simulink model "guidance"  (R2017b)
settings: Solver=FixedStepDiscrete  StartTime=0.0  StopTime=inf  FixedStep=0.01  RelTol=1e-3
model workspace (MAT data in the model file):
  SL_ROS_VariableLengthArrays_MaxSizes.CommonInfo.ArrayTruncateAction = 'EmitWarning'
  SL_ROS_VariableLengthArrays_MaxSizes.MsgTypeMap = containers.Map
  SL_ROS_VariableLengthArrays_MaxSizes.MsgTypeMap.serialization.keys = {'sensor_msgs/Image'}
  SL_ROS_VariableLengthArrays_MaxSizes.MsgTypeMap.serialization.values{1}(1).PropertyName = 'Encoding'
  SL_ROS_VariableLengthArrays_MaxSizes.MsgTypeMap.serialization.values{1}(1).DataType = 'uint8'
  SL_ROS_VariableLengthArrays_MaxSizes.MsgTypeMap.serialization.values{1}(1).MaxLength = 128
  SL_ROS_VariableLengthArrays_MaxSizes.MsgTypeMap.serialization.values{1}(2).PropertyName = 'Data'
  SL_ROS_VariableLengthArrays_MaxSizes.MsgTypeMap.serialization.values{1}(2).DataType = 'uint8'
  SL_ROS_VariableLengthArrays_MaxSizes.MsgTypeMap.serialization.values{1}(2).MaxLength = 921600
  SL_ROS_VariableLengthArrays_MaxSizes.MsgTypeMap.serialization.uniformity = 0
  SL_ROS_VariableLengthArrays_MaxSizes.MsgTypeMap.serialization.keyType = 'char'
  SL_ROS_VariableLengthArrays_MaxSizes.MsgTypeMap.serialization.valueType = 'any'
undefined symbols (not defined in the file): Data, Data_SL_Info
libraries: dspstat3 x13, robotlib x9, simulink x7
settings Model: SimulationMode=external  Creator=a  LastModifiedBy=a
settings OptimizationCC: MaxStackSize=64
settings DebuggingCC: ParameterTunabilityLossMsg=error
settings HardwareCC: ProdBitPerPointer=32  ProdBitPerSizeT=32  ProdBitPerPtrDiffT=32  ProdLargestAtomicInteger=Long  ProdLargestAtomicFloat=Double  ProdWordSize=32  ProdHWDeviceType=ARM Compatible->ARM Cortex
settings SFSimCC: MATLABDynamicMemAlloc=off
settings RTWCC: SystemTargetFile=ert.tlc  HardwareBoard=Robot Operating System (ROS)  TemplateMakefile=ert_default_tmf  GenerateReport=on  Toolchain=Catkin  IncludeHyperlinkInReport=on  LaunchReport=on  TargetLang=C++  GenerateTraceInfo=on  GenerateTraceReport=on  GenerateTraceReportSl=on  GenerateTraceReportSf=on  GenerateTraceReportEml=on
settings CodeAppCC: ForceParamTrailComments=on  IgnoreCustomStorageClasses=off  OperatorAnnotations=on  SimulinkDataObjDesc=on  SFDataObjDesc=on  MATLABFcnDesc=on  InsertBlockDesc=on  StateflowObjectComments=on  MATLABSourceComments=on
settings ERTTargetCC: MultiwordLength=2048  ExtMode=on  ExtModeMexArgs='10.42.0.1' 0 17725
settings SimscapeCC: SimscapeNormalizeSystem=off

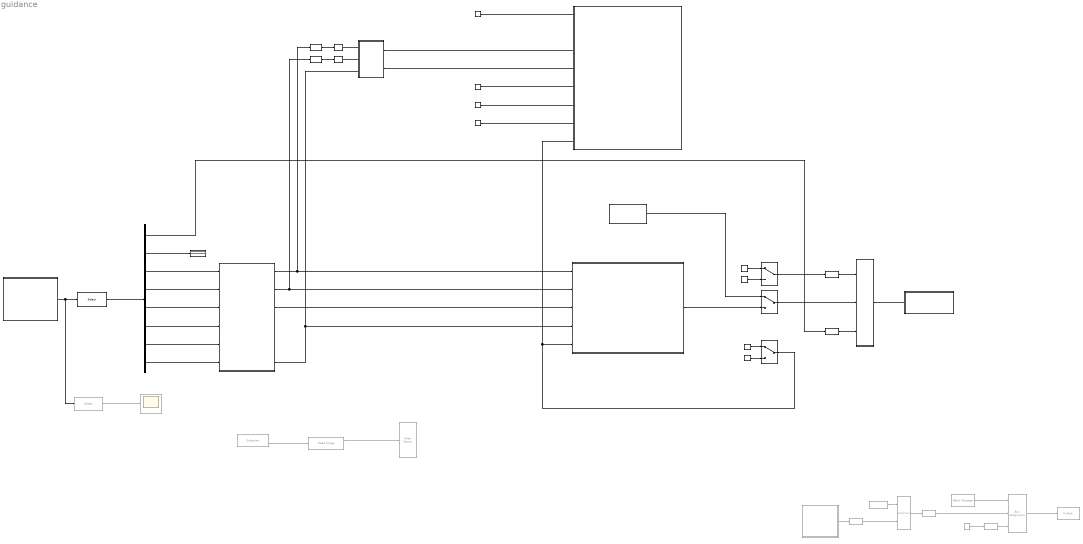
== system guidance ==
  " VX_moving_average" : dspstat3/Moving Average  Method=Sliding window  SpecifyWindowLength=on  WindowLength=5  ForgettingFactor=0.9  SimulateUsing=Code generation
  " VY_moving_average" : dspstat3/Moving Average  Method=Sliding window  SpecifyWindowLength=on  WindowLength=5  ForgettingFactor=0.9  SimulateUsing=Code generation
  Assignment : Assignment  Commented=on  DiagnosticForDimensions=Warning  IndexOptions=Index vector (dialog)  Indices=[1 2 3 4]  OutputSizes=1
  Blank Message : robotlib/Blank Message  Commented=on  SourceLibraryInfo=This block requires Robotics System Toolbox  messageType=std_msgs/Int8MultiArray  SampleTime=0.05
      settings: SourceProductBaseCode=RO
  Bus Assignment : BusAssignment  Commented=on  AssignedSignals=Data,Data_SL_Info.CurrentLength
  Constant1 : Constant  Commented=on  Value=4
  Constant3 : Constant  Commented=on  Value=[1:1:128]
  Data Type Conversion : DataTypeConversion  Commented=on  OutDataTypeStr=double
  Data Type Conversion1 : DataTypeConversion  Commented=on  OutDataTypeStr=uint32
  Data Type Conversion2 : DataTypeConversion  Commented=on  OutDataTypeStr=int8
  Data Type Conversion3 : DataTypeConversion  OutDataTypeStr=single
  Data Type Conversion4 : DataTypeConversion  OutDataTypeStr=single
  Demux : Demux  Outputs=8
  Read Image : robotlib/Read Image  Commented=on  SourceLibraryInfo=This block requires Robotics System Toolbox  MaximumImageSize=[ 320, 240 ]  ImageEncoding=rgb8  ShowAlphaOutput=off  ShowErrorCodeOutput=on  VariableSizeOutputs=off
      settings: SourceProductName=Robotics System Toolbox  SourceProductBaseCode=RO
  Scope : Scope  Commented=on
  Selector : Selector  InputPortWidth=24  IndexOptions=Index vector (dialog)  Indices=[17:24]  OutputSizes=1
  Selector1 : Selector  Commented=on  InputPortWidth=24  IndexOptions=Index vector (dialog)  Indices=[7]  OutputSizes=1
  Subscribe1 : robotlib/Subscribe  Commented=on  SourceLibraryInfo=This block requires Robotics System Toolbox  topicSource=Select from ROS network  topic=/quadrotor_1/image_raw  messageType=sensor_msgs/Image  sampleTime=-1  messageQueueLength=1
      settings: SourceProductBaseCode=RO
  Subsystem : Subsystem  Commented=on  mask{red=0.0, green=0.0, blue=15.0, enable=1}
  Video Viewer : VideoViewer  Commented=on  FigPos=[1 726 1362 626]
  X Derivative : simulink/Discrete/Discrete Derivative  gainval=1.0  ICPrevScaledInput=0.0  OutMin=[]  OutMax=[]  OutDataType=fixdt(1, 16)  OutScaling=2^-10  DoSatur=off
  Y Derivative : simulink/Discrete/Discrete Derivative  gainval=1.0  ICPrevScaledInput=0.0  OutMin=[]  OutMax=[]  OutDataType=fixdt(1, 16)  OutScaling=2^-10  DoSatur=off
  arm : Constant
  arm_disarm_sw : ManualSwitch
  check_arm_status : Subsystem
  command_output : Subsystem
  "command_output " : robotlib/Publish  Commented=on  SourceLibraryInfo=This block requires Robotics System Toolbox  topicSource=Select from ROS network  topic=/quadrotor_1/LED  messageType=std_msgs/Int8MultiArray  messageQueueLength=1
      settings: SourceProductBaseCode=RO
  "data_input " : Subsystem
  disarm : Constant  Value=0
  inertial_to_body_transform : Subsystem
  manual_auto_sw : ManualSwitch
  manual_control : Subsystem  mask{throttle=20.320, roll=0, pitch=0, yaw=0, mode=0}
  mode : Constant  Value=0
  one : Constant
  position_control : Subsystem
  position_filters : Subsystem
  radio_command_frame_rate : Display
  reset_integrator : ManualSwitch
  velocity_control : Subsystem
  vx_setpoint : Constant  Value=0
  vy_setpoint : Constant  Value=0
  yaw_des_rate : Constant  Value=0
  zero : Constant  Value=0
  wires:
  Constant1/1 -> Data Type Conversion1/1
  Data Type Conversion1/1 -> Bus Assignment/3
  Bus Assignment/1 -> "command_output "/1
  Blank Message/1 -> Bus Assignment/1
  Data Type Conversion2/1 -> Bus Assignment/2
  Assignment/1 -> Data Type Conversion2/1
  Data Type Conversion/1 -> Assignment/2
  Constant3/1 -> Assignment/1
  Subsystem/1(Out1) -> Data Type Conversion/1
  disarm/1 -> arm_disarm_sw/1
  check_arm_status/1(Out) -> command_output/1(command)
  Data Type Conversion3/1 -> check_arm_status/3(motors_on)
  Data Type Conversion4/1 -> check_arm_status/1(arm)
  manual_control/1(commands) -> manual_auto_sw/1
  manual_auto_sw/1 -> check_arm_status/2(command)
  arm/1 -> arm_disarm_sw/2
  arm_disarm_sw/1 -> Data Type Conversion4/1
  reset_integrator/1 -> velocity_control/8(Integrator_reset), position_control/5(integrator_reset)
  one/1 -> reset_integrator/2
  zero/1 -> reset_integrator/1
  "data_input "/1(data) -> Selector1/1, Selector/1
  Selector/1 -> Demux/1
  Demux/1 -> Data Type Conversion3/1
  Demux/2 -> radio_command_frame_rate/1
  Subscribe1/2 -> Read Image/1
  Read Image/1 -> Video Viewer/1
  mode/1 -> velocity_control/1(mode)
  Demux/5 -> position_filters/3(z)
  vy_setpoint/1 -> velocity_control/6(vy_setpoint)
  vx_setpoint/1 -> velocity_control/7(vx_setpoint)
  Y Derivative/1 -> " VY_moving_average"/1
  X Derivative/1 -> " VX_moving_average"/1
  Selector1/1 -> Scope/1
  position_filters/1(x_filtered) -> X Derivative/1, position_control/1(X)
  position_filters/6(psi_filtered) -> inertial_to_body_transform/3(PSI), position_control/4(PSI)
  position_filters/2(y_filtered) -> Y Derivative/1, position_control/2(Y)
  Demux/3 -> position_filters/1(x)
  Demux/4 -> position_filters/2(y)
  Demux/6 -> position_filters/4(phi)
  Demux/7 -> position_filters/5(theta)
  Demux/8 -> position_filters/6(psi)
  position_filters/3(z_filtered) -> position_control/3(Z)
  inertial_to_body_transform/1(vx) -> velocity_control/3(vx)
  inertial_to_body_transform/2(vy) -> velocity_control/4(vy)
  " VX_moving_average"/1 -> inertial_to_body_transform/1(VX)
  " VY_moving_average"/1 -> inertial_to_body_transform/2(VY)
  position_control/1(radio_command) -> manual_auto_sw/2
  yaw_des_rate/1 -> velocity_control/5(yaw_des_rate)

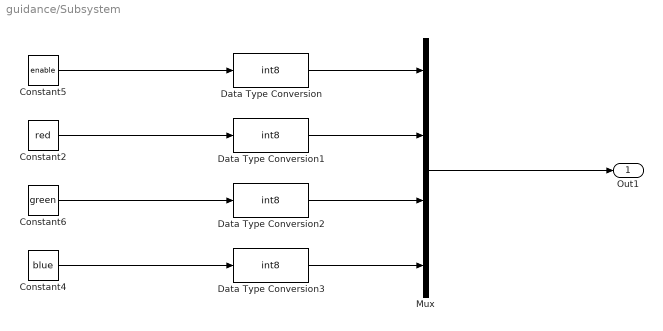
== system guidance/Subsystem ==
  Constant2 : Constant  Value=red
  Constant4 : Constant  Value=blue
  Constant5 : Constant  Value=enable
  Constant6 : Constant  Value=green
  Data Type Conversion{,1..3} (4 alike) : DataTypeConversion  OutDataTypeStr=int8
  Mux : Mux
  Out1 : Outport
  wires:
  Constant2/1 -> Data Type Conversion1/1
  Mux/1 -> Out1/1
  Constant5/1 -> Data Type Conversion/1
  Constant4/1 -> Data Type Conversion3/1
  Constant6/1 -> Data Type Conversion2/1
  Data Type Conversion/1 -> Mux/1
  Data Type Conversion1/1 -> Mux/2
  Data Type Conversion2/1 -> Mux/3
  Data Type Conversion3/1 -> Mux/4

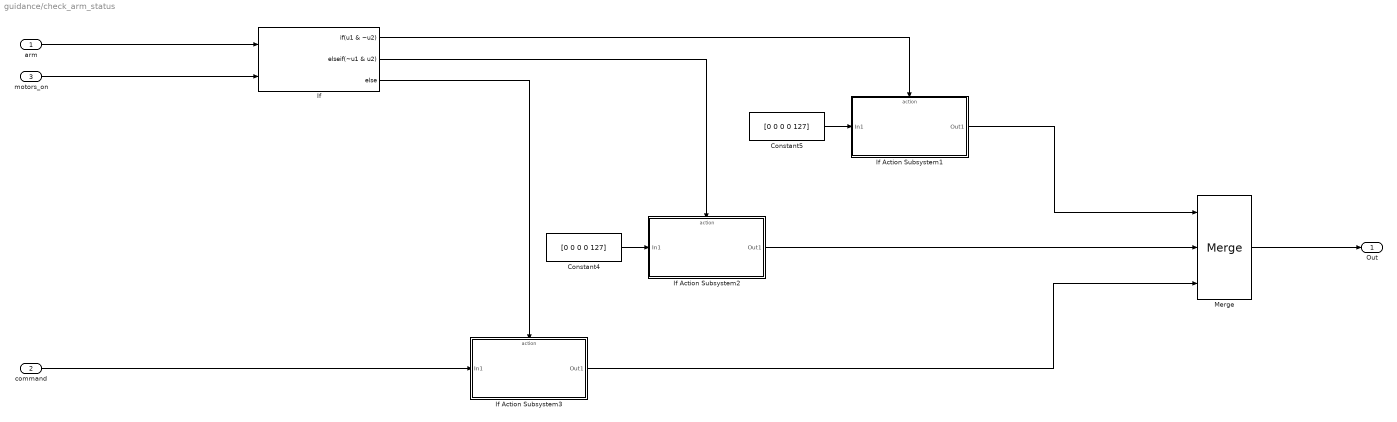
== system guidance/check_arm_status ==
  arm : Inport
  command : Inport  Port=2
  motors_on : Inport  Port=3
  Constant4 : Constant  Value=[0 0 0 0 127]
  Constant5 : Constant  Value=[0 0 0 0 127]
  If : If  NumInputs=2  IfExpression=u1 & ~u2  ElseIfExpressions=~u1 & u2
  If Action Subsystem1 : Subsystem  TreatAsAtomicUnit=on
  If Action Subsystem2 : Subsystem  TreatAsAtomicUnit=on
  If Action Subsystem3 : Subsystem  TreatAsAtomicUnit=on
  Merge : Merge  Inputs=3
  Out : Outport
  wires:
  If/1 -> If Action Subsystem1/Action
  Constant4/1 -> If Action Subsystem2/1(In1)
  If/3 -> If Action Subsystem3/Action
  Constant5/1 -> If Action Subsystem1/1(In1)
  If/2 -> If Action Subsystem2/Action
  If Action Subsystem2/1(Out1) -> Merge/2
  motors_on/1 -> If/2
  command/1 -> If Action Subsystem3/1(In1)
  If Action Subsystem1/1(Out1) -> Merge/1
  If Action Subsystem3/1(Out1) -> Merge/3
  arm/1 -> If/1
  Merge/1 -> Out/1

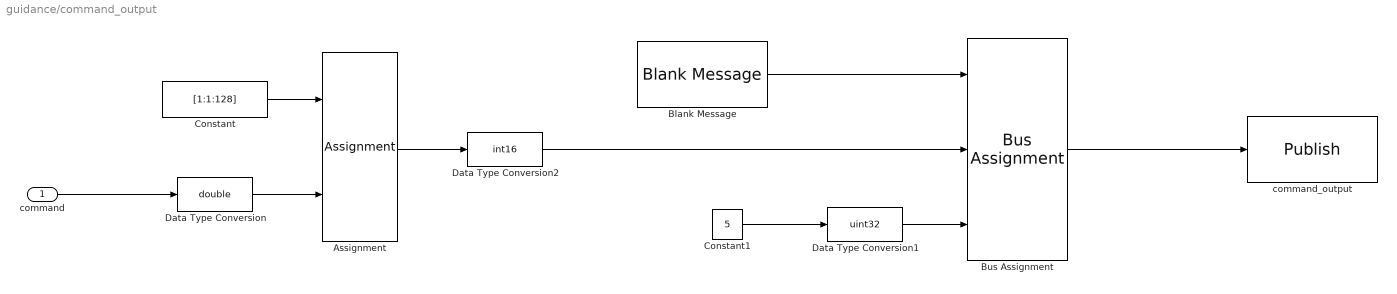
== system guidance/command_output ==
  command : Inport
  Assignment : Assignment  DiagnosticForDimensions=Warning  IndexOptions=Index vector (dialog)  Indices=[1 2 3 4 5]  OutputSizes=1
  Blank Message : robotlib/Blank Message  SourceLibraryInfo=This block requires Robotics System Toolbox  messageType=std_msgs/Int16MultiArray  SampleTime=inf
      settings: SourceProductBaseCode=RO
  Bus Assignment : BusAssignment  AssignedSignals=Data,Data_SL_Info.CurrentLength
  Constant : Constant  Value=[1:1:128]
  Constant1 : Constant  Value=5
  Data Type Conversion : DataTypeConversion  OutDataTypeStr=double
  Data Type Conversion1 : DataTypeConversion  OutDataTypeStr=uint32
  Data Type Conversion2 : DataTypeConversion  OutDataTypeStr=int16
  "command_output " : robotlib/Publish  SourceLibraryInfo=This block requires Robotics System Toolbox  topicSource=Select from ROS network  topic=/quadrotor_1/rpyt_command  messageType=std_msgs/Int16MultiArray  messageQueueLength=1
      settings: SourceProductBaseCode=RO
  wires:
  Constant1/1 -> Data Type Conversion1/1
  Data Type Conversion1/1 -> Bus Assignment/3
  Bus Assignment/1 -> "command_output "/1
  Data Type Conversion2/1 -> Bus Assignment/2
  Assignment/1 -> Data Type Conversion2/1
  Blank Message/1 -> Bus Assignment/1
  Data Type Conversion/1 -> Assignment/2
  command/1 -> Data Type Conversion/1
  Constant/1 -> Assignment/1

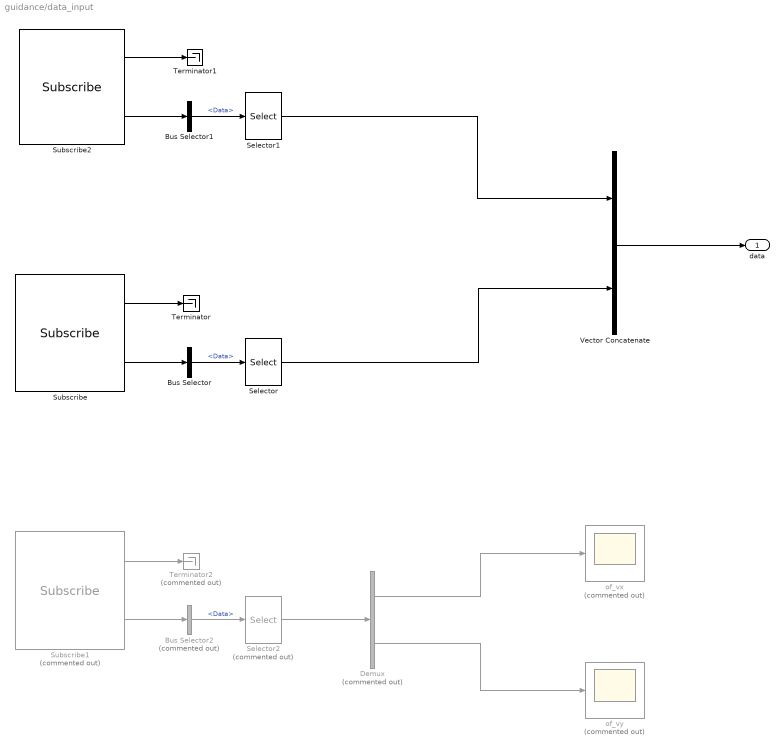
== system guidance/data_input  ==
  Bus Selector : BusSelector  OutputSignals=Data
  Bus Selector1 : BusSelector  OutputSignals=Data
  Bus Selector2 : BusSelector  Commented=on  OutputSignals=Data
  Demux : Demux  Commented=on  Outputs=2
  Selector : Selector  InputPortWidth=128  IndexOptions=Index vector (dialog)  Indices=[1 2 3 4 5 6]  OutputSizes=1
  Selector1 : Selector  InputPortWidth=128  IndexOptions=Index vector (dialog)  Indices=[1 2 3 4 5 6 7 8 9 10 11 12 13 14 15 16 17 18]  OutputSizes=1
  Selector2 : Selector  Commented=on  InputPortWidth=128  IndexOptions=Index vector (dialog)  Indices=[1 2]  OutputSizes=1
  Subscribe : robotlib/Subscribe  SourceLibraryInfo=This block requires Robotics System Toolbox  topicSource=Select from ROS network  topic=/quadrotor_1/nav  messageType=std_msgs/Float32MultiArray  sampleTime=-1  messageQueueLength=1
      settings: SourceProductBaseCode=RO
  Subscribe1 : robotlib/Subscribe  Commented=on  SourceLibraryInfo=This block requires Robotics System Toolbox  topicSource=Select from ROS network  topic=/quadrotor_1/optical_flow  messageType=std_msgs/Float32MultiArray  sampleTime=-1  messageQueueLength=1
      settings: SourceProductBaseCode=RO
  Subscribe2 : robotlib/Subscribe  SourceLibraryInfo=This block requires Robotics System Toolbox  topicSource=Select from ROS network  topic=/quadrotor_1/sensor_data  messageType=std_msgs/Float32MultiArray  sampleTime=-1  messageQueueLength=1
      settings: SourceProductBaseCode=RO
  Terminator : Terminator
  Terminator1 : Terminator
  Terminator2 : Terminator  Commented=on
  Vector Concatenate : Concatenate
  of_vx : Scope  Commented=on
  of_vy : Scope  Commented=on
  data : Outport
  wires:
  Subscribe/1 -> Terminator/1
  Selector/1 -> Vector Concatenate/2
  Subscribe2/1 -> Terminator1/1
  Subscribe2/2 -> Bus Selector1/1
  Subscribe/2 -> Bus Selector/1
  Bus Selector/1 -> Selector/1  "<Data>"
  Bus Selector1/1 -> Selector1/1  "<Data>"
  Selector1/1 -> Vector Concatenate/1
  Vector Concatenate/1 -> data/1
  Subscribe1/2 -> Bus Selector2/1
  Subscribe1/1 -> Terminator2/1
  Bus Selector2/1 -> Selector2/1  "<Data>"
  Selector2/1 -> Demux/1
  Demux/1 -> of_vx/1
  Demux/2 -> of_vy/1

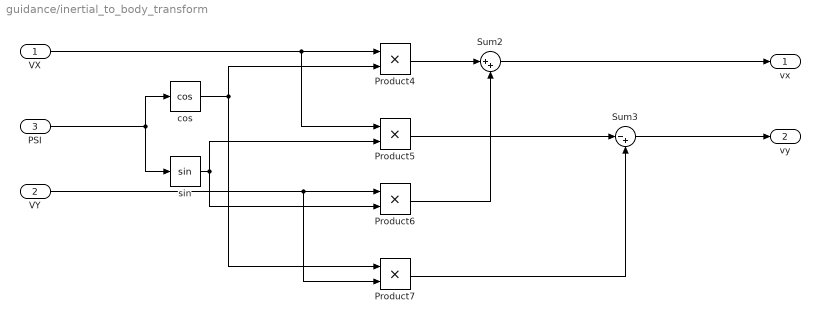
== system guidance/inertial_to_body_transform ==
  VX : Inport
  VY : Inport  Port=2
  PSI : Inport  Port=3
  Product{4..7} (4 alike) : Product
  Sum2 : Sum  Inputs=|++
  Sum3 : Sum  Inputs=|-+
  cos : Trigonometry  Operator=cos
  sin : Trigonometry
  vx : Outport
  vy : Outport  Port=2
  wires:
  Product5/1 -> Sum3/1
  PSI/1 -> sin/1, cos/1
  cos/1 -> Product7/1, Product4/2
  VY/1 -> Product7/2, Product6/1
  Sum3/1 -> vy/1
  sin/1 -> Product6/2, Product5/2
  VX/1 -> Product5/1, Product4/1
  Product6/1 -> Sum2/2
  Product7/1 -> Sum3/2
  Sum2/1 -> vx/1
  Product4/1 -> Sum2/1

== system guidance/manual_control ==
  Constant : Constant  Value=[mode throttle roll pitch yaw]
  commands : Outport
  wires:
  Constant/1 -> commands/1

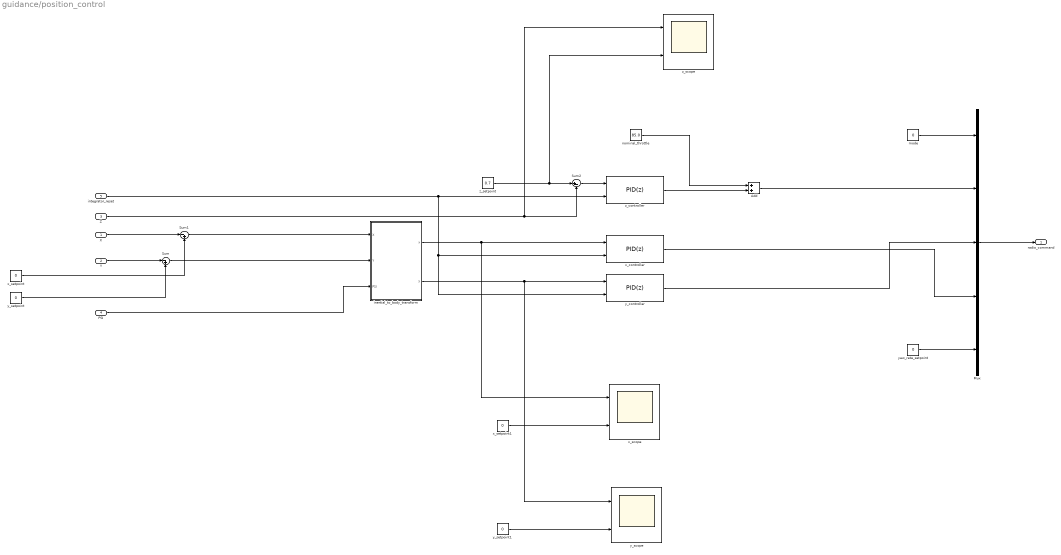
== system guidance/position_control ==
  X : Inport
  Y : Inport  Port=2
  Z : Inport  Port=3
  PSI : Inport  Port=4
  integrator_reset : Inport  Port=5
  Add : Sum
  Mux : Mux  Inputs=5
  Sum : Sum  Inputs=|-+
  Sum1 : Sum  Inputs=|-+
  Sum2 : Sum  Inputs=|+-
  inertial_to_body_transform : Subsystem
  mode : Constant  Value=0
  nominal_throttle : Constant  Value=85.0
  x_controller : simulink/Continuous/PID Controller  Controller=PID  TimeDomain=Discrete-time  SampleTime=-1  IntegratorMethod=Forward Euler  FilterMethod=Forward Euler  Form=Parallel  UseFilter=on  ControllerParametersSource=internal  P=10  I=0  D=0  N=100  InitialConditionSource=internal  InitialConditionForIntegrator=0  InitialConditionForFilter=0  ExternalReset=either  LimitOutput=on  UpperSaturationLimit=1.5  LowerSaturationLimit=-1.5  LinearizeAsGain=off  AntiWindupMode=none  Kb=1  TrackingMode=off  Kt=1  PParamMin=[]  PParamMax=[]  IParamMin=[]  IParamMax=[]  DParamMin=[]  DParamMax=[]  NParamMin=[]  NParamMax=[]  KbParamMin=[]  KbParamMax=[]  KtParamMin=[]  KtParamMax=[]  POutMin=[]  POutMax=[]  IOutMin=[]  IOutMax=[]  DOutMin=[]  DOutMax=[]  NOutMin=[]  NOutMax=[]  KbOutMin=[]  KbOutMax=[]  KtOutMin=[]  KtOutMax=[]  IntegratorOutMin=[]  IntegratorOutMax=[]  FilterOutMin=[]  FilterOutMax=[]  SumOutMin=[]  SumOutMax=[]  SumI1OutMin=[]  SumI1OutMax=[]  SumI2OutMin=[]  SumI2OutMax=[]  SumI3OutMin=[]  SumI3OutMax=[]  SumDOutMin=[]  SumDOutMax=[]  SaturationOutMin=[]  SaturationOutMax=[]  IntegratorContinuousStateAttributes=''  IntegratorStateMustResolveToSignalObject=off  IntegratorRTWStateStorageClass=Auto  FilterContinuousStateAttributes=''  FilterStateMustResolveToSignalObject=off  FilterRTWStateStorageClass=Auto  DifferentiatorICPrevScaledInput=0  DifferentiatorOutMin=[]  DifferentiatorOutMax=[]  InitialConditionSetting=State (most efficient)  FilterDiffOutCoefMin=[]  FilterDiffOutCoefMax=[]  SumDenOutMin=[]  SumDenOutMax=[]  SumNumOutMin=[]  SumNumOutMax=[]  ReciprocalOutMin=[]  ReciprocalOutMax=[]  DivideOutMin=[]  DivideOutMax=[]  TunerSelectOption=Transfer Function Based (PID Tuner App)
  x_scope : Scope  NumInputPorts=2
  x_setpoint : Constant  Value=0
  x_setpoint1 : Constant  Value=0
  y_controller : simulink/Continuous/PID Controller  Controller=PID  TimeDomain=Discrete-time  SampleTime=-1  IntegratorMethod=Forward Euler  FilterMethod=Forward Euler  Form=Parallel  UseFilter=on  ControllerParametersSource=internal  P=10  I=0  D=0  N=100  InitialConditionSource=internal  InitialConditionForIntegrator=0  InitialConditionForFilter=0  ExternalReset=either  LimitOutput=on  UpperSaturationLimit=1.5  LowerSaturationLimit=-1.5  LinearizeAsGain=off  AntiWindupMode=none  Kb=1  TrackingMode=off  Kt=1  PParamMin=[]  PParamMax=[]  IParamMin=[]  IParamMax=[]  DParamMin=[]  DParamMax=[]  NParamMin=[]  NParamMax=[]  KbParamMin=[]  KbParamMax=[]  KtParamMin=[]  KtParamMax=[]  POutMin=[]  POutMax=[]  IOutMin=[]  IOutMax=[]  DOutMin=[]  DOutMax=[]  NOutMin=[]  NOutMax=[]  KbOutMin=[]  KbOutMax=[]  KtOutMin=[]  KtOutMax=[]  IntegratorOutMin=[]  IntegratorOutMax=[]  FilterOutMin=[]  FilterOutMax=[]  SumOutMin=[]  SumOutMax=[]  SumI1OutMin=[]  SumI1OutMax=[]  SumI2OutMin=[]  SumI2OutMax=[]  SumI3OutMin=[]  SumI3OutMax=[]  SumDOutMin=[]  SumDOutMax=[]  SaturationOutMin=[]  SaturationOutMax=[]  IntegratorContinuousStateAttributes=''  IntegratorStateMustResolveToSignalObject=off  IntegratorRTWStateStorageClass=Auto  FilterContinuousStateAttributes=''  FilterStateMustResolveToSignalObject=off  FilterRTWStateStorageClass=Auto  DifferentiatorICPrevScaledInput=0  DifferentiatorOutMin=[]  DifferentiatorOutMax=[]  InitialConditionSetting=State (most efficient)  FilterDiffOutCoefMin=[]  FilterDiffOutCoefMax=[]  SumDenOutMin=[]  SumDenOutMax=[]  SumNumOutMin=[]  SumNumOutMax=[]  ReciprocalOutMin=[]  ReciprocalOutMax=[]  DivideOutMin=[]  DivideOutMax=[]  TunerSelectOption=Transfer Function Based (PID Tuner App)
  y_scope : Scope  NumInputPorts=2
  y_setpoint : Constant  Value=0
  y_setpoint1 : Constant  Value=0
  yaw_rate_setpoint : Constant  Value=0
  z_controller : simulink/Continuous/PID Controller  Controller=PID  TimeDomain=Discrete-time  SampleTime=-1  IntegratorMethod=Forward Euler  FilterMethod=Forward Euler  Form=Parallel  UseFilter=on  ControllerParametersSource=internal  P=20  I=10  D=14  N=100  InitialConditionSource=internal  InitialConditionForIntegrator=0  InitialConditionForFilter=0  ExternalReset=either  LimitOutput=on  UpperSaturationLimit=35  LowerSaturationLimit=-85  LinearizeAsGain=off  AntiWindupMode=none  Kb=1  TrackingMode=off  Kt=1  PParamMin=[]  PParamMax=[]  IParamMin=[]  IParamMax=[]  DParamMin=[]  DParamMax=[]  NParamMin=[]  NParamMax=[]  KbParamMin=[]  KbParamMax=[]  KtParamMin=[]  KtParamMax=[]  POutMin=[]  POutMax=[]  IOutMin=[]  IOutMax=[]  DOutMin=[]  DOutMax=[]  NOutMin=[]  NOutMax=[]  KbOutMin=[]  KbOutMax=[]  KtOutMin=[]  KtOutMax=[]  IntegratorOutMin=[]  IntegratorOutMax=[]  FilterOutMin=[]  FilterOutMax=[]  SumOutMin=[]  SumOutMax=[]  SumI1OutMin=[]  SumI1OutMax=[]  SumI2OutMin=[]  SumI2OutMax=[]  SumI3OutMin=[]  SumI3OutMax=[]  SumDOutMin=[]  SumDOutMax=[]  SaturationOutMin=[]  SaturationOutMax=[]  IntegratorContinuousStateAttributes=''  IntegratorStateMustResolveToSignalObject=off  IntegratorRTWStateStorageClass=Auto  FilterContinuousStateAttributes=''  FilterStateMustResolveToSignalObject=off  FilterRTWStateStorageClass=Auto  DifferentiatorICPrevScaledInput=0  DifferentiatorOutMin=[]  DifferentiatorOutMax=[]  InitialConditionSetting=State (most efficient)  FilterDiffOutCoefMin=[]  FilterDiffOutCoefMax=[]  SumDenOutMin=[]  SumDenOutMax=[]  SumNumOutMin=[]  SumNumOutMax=[]  ReciprocalOutMin=[]  ReciprocalOutMax=[]  DivideOutMin=[]  DivideOutMax=[]  TunerSelectOption=Transfer Function Based (PID Tuner App)
  z_scope : Scope  NumInputPorts=2
  z_setpoint : Constant  Value=0.7
  radio_command : Outport
  wires:
  Z/1 -> z_scope/1, Sum2/2
  nominal_throttle/1 -> Add/1
  z_controller/1 -> Add/2
  Sum2/1 -> z_controller/1
  z_setpoint/1 -> z_scope/2, Sum2/1
  integrator_reset/1 -> y_controller/2, x_controller/2, z_controller/2
  Y/1 -> Sum/1
  X/1 -> Sum1/1
  yaw_rate_setpoint/1 -> Mux/5
  y_controller/1 -> Mux/3
  PSI/1 -> inertial_to_body_transform/3(PSI)
  x_controller/1 -> Mux/4
  y_setpoint/1 -> Sum/2
  Sum/1 -> inertial_to_body_transform/2(Y)
  Sum1/1 -> inertial_to_body_transform/1(X)
  x_setpoint/1 -> Sum1/2
  inertial_to_body_transform/1(x) -> x_scope/1, x_controller/1
  inertial_to_body_transform/2(y) -> y_scope/1, y_controller/1
  Add/1 -> Mux/2
  mode/1 -> Mux/1
  Mux/1 -> radio_command/1
  x_setpoint1/1 -> x_scope/2
  y_setpoint1/1 -> y_scope/2

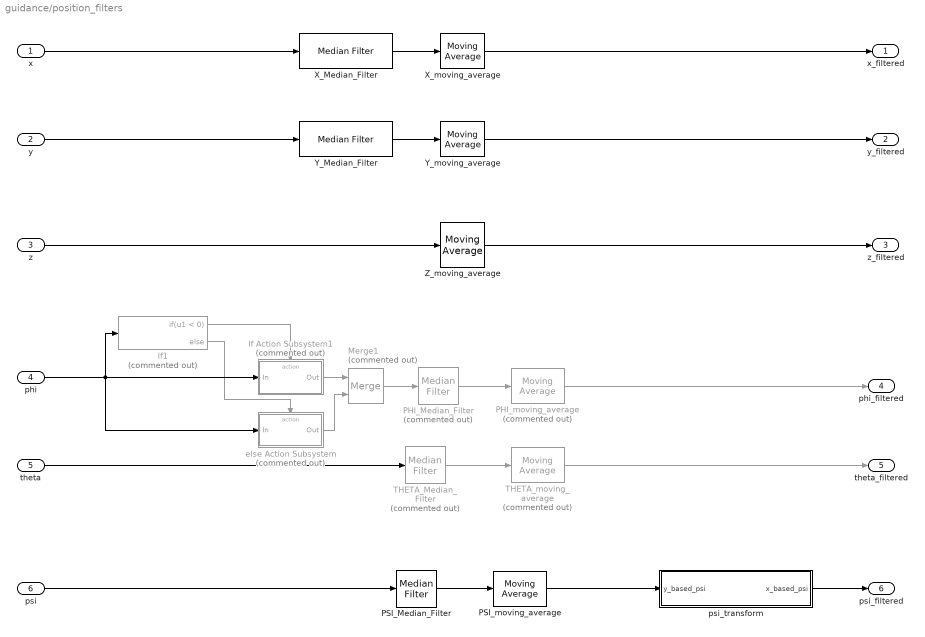
== system guidance/position_filters ==
  x : Inport
  y : Inport  Port=2
  z : Inport  Port=3
  phi : Inport  Port=4
  theta : Inport  Port=5
  psi : Inport  Port=6
  " PHI_moving_average" : dspstat3/Moving Average  Commented=on  Method=Sliding window  SpecifyWindowLength=on  WindowLength=30  ForgettingFactor=0.9  SimulateUsing=Code generation
  " PSI_moving_average" : dspstat3/Moving Average  Method=Sliding window  SpecifyWindowLength=on  WindowLength=30  ForgettingFactor=0.9  SimulateUsing=Code generation
  " THETA_moving_average" : dspstat3/Moving Average  Commented=on  Method=Sliding window  SpecifyWindowLength=on  WindowLength=30  ForgettingFactor=0.9  SimulateUsing=Code generation
  " X_moving_average" : dspstat3/Moving Average  Method=Sliding window  SpecifyWindowLength=on  WindowLength=30  ForgettingFactor=0.9  SimulateUsing=Code generation
  " Y_moving_average" : dspstat3/Moving Average  Method=Sliding window  SpecifyWindowLength=on  WindowLength=30  ForgettingFactor=0.9  SimulateUsing=Code generation
  If Action Subsystem1 : Subsystem  Commented=on  TreatAsAtomicUnit=on
  If1 : If  Commented=on  IfExpression=u1 < 0
  Merge1 : Merge  Commented=on
  PHI_Median_Filter : dspstat3/Median Filter  Commented=on  WindowLength=10  SimulateUsing=Interpreted execution
      settings: SourceProductName=DSP System Toolbox  SourceProductBaseCode=DS
  PSI_Median_Filter : dspstat3/Median Filter  WindowLength=10  SimulateUsing=Interpreted execution
      settings: SourceProductName=DSP System Toolbox  SourceProductBaseCode=DS
  THETA_Median_Filter : dspstat3/Median Filter  Commented=on  WindowLength=10  SimulateUsing=Interpreted execution
      settings: SourceProductName=DSP System Toolbox  SourceProductBaseCode=DS
  X_Median_Filter : dspstat3/Median Filter  WindowLength=10  SimulateUsing=Interpreted execution
      settings: SourceProductName=DSP System Toolbox  SourceProductBaseCode=DS
  Y_Median_Filter : dspstat3/Median Filter  WindowLength=10  SimulateUsing=Interpreted execution
      settings: SourceProductName=DSP System Toolbox  SourceProductBaseCode=DS
  Z_moving_average : dspstat3/Moving Average  Method=Sliding window  SpecifyWindowLength=on  WindowLength=20  ForgettingFactor=0.9  SimulateUsing=Code generation
  else Action Subsystem : Subsystem  Commented=on  TreatAsAtomicUnit=on
  psi_transform : Subsystem
  x_filtered : Outport
  y_filtered : Outport  Port=2
  z_filtered : Outport  Port=3
  phi_filtered : Outport  Port=4
  theta_filtered : Outport  Port=5
  psi_filtered : Outport  Port=6
  wires:
  psi/1 -> PSI_Median_Filter/1
  x/1 -> X_Median_Filter/1
  y/1 -> Y_Median_Filter/1
  Y_Median_Filter/1 -> " Y_moving_average"/1
  THETA_Median_Filter/1 -> " THETA_moving_average"/1
  else Action Subsystem/1(Out) -> Merge1/2
  PSI_Median_Filter/1 -> " PSI_moving_average"/1
  " Y_moving_average"/1 -> y_filtered/1
  If Action Subsystem1/1(Out) -> Merge1/1
  " X_moving_average"/1 -> x_filtered/1
  " THETA_moving_average"/1 -> theta_filtered/1
  X_Median_Filter/1 -> " X_moving_average"/1
  psi_transform/1(x_based_psi) -> psi_filtered/1
  " PSI_moving_average"/1 -> psi_transform/1(y_based_psi)
  If1/2 -> else Action Subsystem/Action
  phi/1 -> If1/1, else Action Subsystem/1(In), If Action Subsystem1/1(In)
  theta/1 -> THETA_Median_Filter/1
  " PHI_moving_average"/1 -> phi_filtered/1
  PHI_Median_Filter/1 -> " PHI_moving_average"/1
  If1/1 -> If Action Subsystem1/Action
  Merge1/1 -> PHI_Median_Filter/1
  z/1 -> Z_moving_average/1
  Z_moving_average/1 -> z_filtered/1

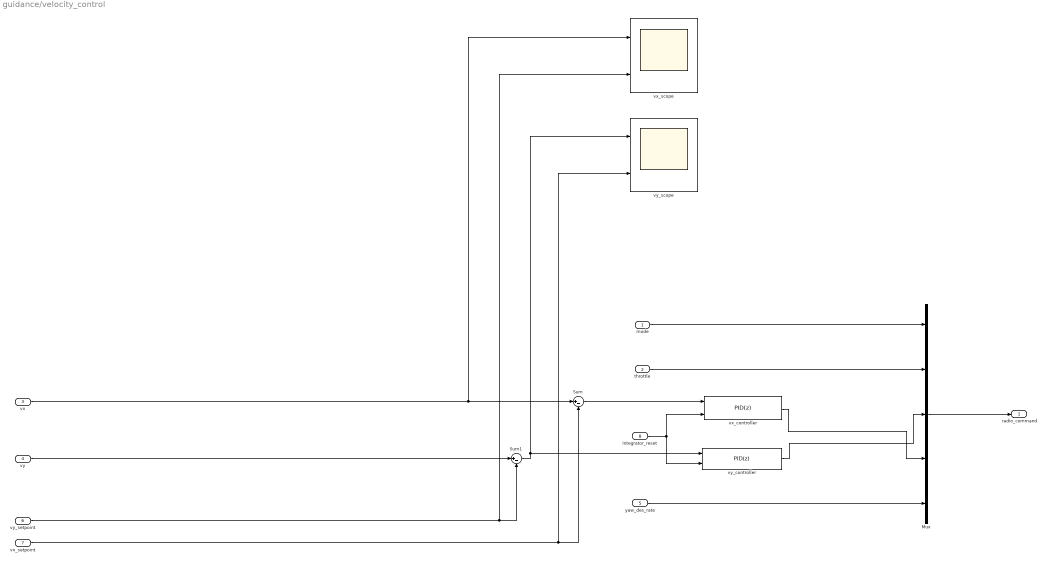
== system guidance/velocity_control ==
  mode : Inport
  throttle : Inport  Port=2
  vx : Inport  Port=3
  vy : Inport  Port=4
  yaw_des_rate : Inport  Port=5
  vy_setpoint : Inport  Port=6
  vx_setpoint : Inport  Port=7
  Integrator_reset : Inport  Port=8
  Mux : Mux  Inputs=5
  Sum : Sum  Inputs=|+-
  Sum1 : Sum  Inputs=|+-
  vx_controller : simulink/Continuous/PID Controller  Controller=PID  TimeDomain=Discrete-time  SampleTime=-1  IntegratorMethod=Forward Euler  FilterMethod=Forward Euler  Form=Parallel  UseFilter=on  ControllerParametersSource=internal  P=35  I=30  D=4  N=100  InitialConditionSource=internal  InitialConditionForIntegrator=0  InitialConditionForFilter=0  ExternalReset=either  LimitOutput=on  UpperSaturationLimit=127  LowerSaturationLimit=-127  LinearizeAsGain=off  AntiWindupMode=none  Kb=1  TrackingMode=off  Kt=1  PParamMin=[]  PParamMax=[]  IParamMin=[]  IParamMax=[]  DParamMin=[]  DParamMax=[]  NParamMin=[]  NParamMax=[]  KbParamMin=[]  KbParamMax=[]  KtParamMin=[]  KtParamMax=[]  POutMin=[]  POutMax=[]  IOutMin=[]  IOutMax=[]  DOutMin=[]  DOutMax=[]  NOutMin=[]  NOutMax=[]  KbOutMin=[]  KbOutMax=[]  KtOutMin=[]  KtOutMax=[]  IntegratorOutMin=[]  IntegratorOutMax=[]  FilterOutMin=[]  FilterOutMax=[]  SumOutMin=[]  SumOutMax=[]  SumI1OutMin=[]  SumI1OutMax=[]  SumI2OutMin=[]  SumI2OutMax=[]  SumI3OutMin=[]  SumI3OutMax=[]  SumDOutMin=[]  SumDOutMax=[]  SaturationOutMin=[]  SaturationOutMax=[]  IntegratorContinuousStateAttributes=''  IntegratorStateMustResolveToSignalObject=off  IntegratorRTWStateStorageClass=Auto  FilterContinuousStateAttributes=''  FilterStateMustResolveToSignalObject=off  FilterRTWStateStorageClass=Auto  DifferentiatorICPrevScaledInput=0  DifferentiatorOutMin=[]  DifferentiatorOutMax=[]  InitialConditionSetting=State (most efficient)  FilterDiffOutCoefMin=[]  FilterDiffOutCoefMax=[]  SumDenOutMin=[]  SumDenOutMax=[]  SumNumOutMin=[]  SumNumOutMax=[]  ReciprocalOutMin=[]  ReciprocalOutMax=[]  DivideOutMin=[]  DivideOutMax=[]  TunerSelectOption=Transfer Function Based (PID Tuner App)
  vx_scope : Scope  NumInputPorts=2
  vy_controller : simulink/Continuous/PID Controller  Controller=PID  TimeDomain=Discrete-time  SampleTime=-1  IntegratorMethod=Forward Euler  FilterMethod=Forward Euler  Form=Parallel  UseFilter=on  ControllerParametersSource=internal  P=40  I=30  D=10  N=100  InitialConditionSource=internal  InitialConditionForIntegrator=0  InitialConditionForFilter=0  ExternalReset=either  LimitOutput=on  UpperSaturationLimit=127  LowerSaturationLimit=-127  LinearizeAsGain=off  AntiWindupMode=none  Kb=1  TrackingMode=off  Kt=1  PParamMin=[]  PParamMax=[]  IParamMin=[]  IParamMax=[]  DParamMin=[]  DParamMax=[]  NParamMin=[]  NParamMax=[]  KbParamMin=[]  KbParamMax=[]  KtParamMin=[]  KtParamMax=[]  POutMin=[]  POutMax=[]  IOutMin=[]  IOutMax=[]  DOutMin=[]  DOutMax=[]  NOutMin=[]  NOutMax=[]  KbOutMin=[]  KbOutMax=[]  KtOutMin=[]  KtOutMax=[]  IntegratorOutMin=[]  IntegratorOutMax=[]  FilterOutMin=[]  FilterOutMax=[]  SumOutMin=[]  SumOutMax=[]  SumI1OutMin=[]  SumI1OutMax=[]  SumI2OutMin=[]  SumI2OutMax=[]  SumI3OutMin=[]  SumI3OutMax=[]  SumDOutMin=[]  SumDOutMax=[]  SaturationOutMin=[]  SaturationOutMax=[]  IntegratorContinuousStateAttributes=''  IntegratorStateMustResolveToSignalObject=off  IntegratorRTWStateStorageClass=Auto  FilterContinuousStateAttributes=''  FilterStateMustResolveToSignalObject=off  FilterRTWStateStorageClass=Auto  DifferentiatorICPrevScaledInput=0  DifferentiatorOutMin=[]  DifferentiatorOutMax=[]  InitialConditionSetting=State (most efficient)  FilterDiffOutCoefMin=[]  FilterDiffOutCoefMax=[]  SumDenOutMin=[]  SumDenOutMax=[]  SumNumOutMin=[]  SumNumOutMax=[]  ReciprocalOutMin=[]  ReciprocalOutMax=[]  DivideOutMin=[]  DivideOutMax=[]  TunerSelectOption=Transfer Function Based (PID Tuner App)
  vy_scope : Scope  NumInputPorts=2
  radio_command : Outport
  wires:
  vy/1 -> Sum1/1
  vy_setpoint/1 -> vx_scope/2, Sum1/2
  Sum1/1 -> vy_controller/1, vy_scope/1
  vy_controller/1 -> Mux/3
  Mux/1 -> radio_command/1
  vx/1 -> vx_scope/1, Sum/1
  Sum/1 -> vx_controller/1
  vx_setpoint/1 -> vy_scope/2, Sum/2
  mode/1 -> Mux/1
  yaw_des_rate/1 -> Mux/5
  throttle/1 -> Mux/2
  vx_controller/1 -> Mux/4
  Integrator_reset/1 -> vy_controller/2, vx_controller/2

== system guidance/check_arm_status/If Action Subsystem1 ==
  In1 : Inport
  Action Port : ActionPort  ActionType=then
  Out1 : Outport
  wires:
  In1/1 -> Out1/1

== system guidance/check_arm_status/If Action Subsystem2 ==
  In1 : Inport
  Action Port : ActionPort  ActionType=elseif
  Out1 : Outport
  wires:
  In1/1 -> Out1/1

== system guidance/check_arm_status/If Action Subsystem3 ==
  In1 : Inport
  Action Port : ActionPort  ActionType=else
  Out1 : Outport
  wires:
  In1/1 -> Out1/1

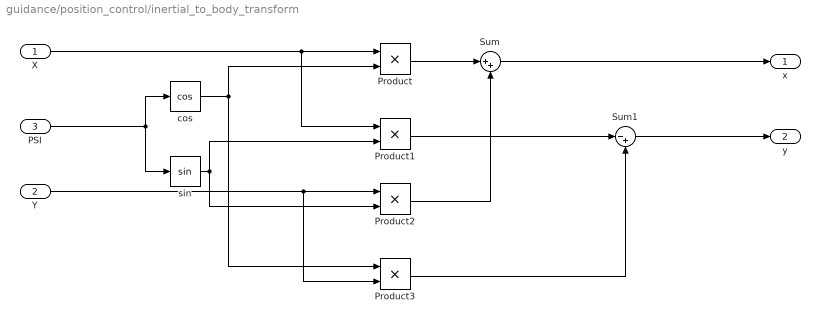
== system guidance/position_control/inertial_to_body_transform ==
  X : Inport
  Y : Inport  Port=2
  PSI : Inport  Port=3
  Product{,1..3} (4 alike) : Product
  Sum : Sum  Inputs=|++
  Sum1 : Sum  Inputs=|-+
  cos : Trigonometry  Operator=cos
  sin : Trigonometry
  x : Outport
  y : Outport  Port=2
  wires:
  sin/1 -> Product2/2, Product1/2
  Product3/1 -> Sum1/2
  Sum/1 -> x/1
  Product/1 -> Sum/1
  Y/1 -> Product3/2, Product2/1
  PSI/1 -> sin/1, cos/1
  X/1 -> Product1/1, Product/1
  Sum1/1 -> y/1
  cos/1 -> Product3/1, Product/2
  Product2/1 -> Sum/2
  Product1/1 -> Sum1/1

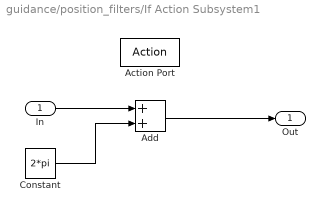
== system guidance/position_filters/If Action Subsystem1 ==
  In : Inport
  Action Port : ActionPort  ActionType=then
  Add : Sum
  Constant : Constant  Value=2*pi
  Out : Outport
  wires:
  Constant/1 -> Add/2
  Add/1 -> Out/1
  In/1 -> Add/1

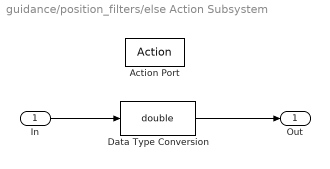
== system guidance/position_filters/else Action Subsystem ==
  In : Inport
  Action Port : ActionPort  ActionType=else
  Data Type Conversion : DataTypeConversion  OutDataTypeStr=double
  Out : Outport
  wires:
  Data Type Conversion/1 -> Out/1
  In/1 -> Data Type Conversion/1

== system guidance/position_filters/psi_transform ==
  y_based_psi : Inport
  Add : Sum
  additional : Constant  Value=90
  x_based_psi : Outport
  wires:
  y_based_psi/1 -> Add/2
  Add/1 -> x_based_psi/1
  additional/1 -> Add/1
